simulink model "simplified_sim_for_linearize"  (R2024b)
settings: Solver=VariableStepAuto  StartTime=0.0  StopTime=15  FixedStep=0.05  MaxStep=0.2  RelTol=1e-3
values from neighbouring files (symbols this model uses):
  AfoilA = 0.046    [model_parameters.m]
  AfoilFP = 0.048    [model_parameters.m]
  AfoilFS = 0.048    [model_parameters.m]
  alpha0012 = data0012(:,1)    [model_parameters.m]
  alpha63412wing = data63412wing(:,1)    [model_parameters.m]
  cd0012 = data0012(:,3)    [model_parameters.m]
  cdi63412wing = data63412wing(:,4)    [model_parameters.m]
  cdv63412wing = data63412wing(:,5)    [model_parameters.m]
  cl63412wing = data63412wing(:,3)    [model_parameters.m]
  cm63412wing = data63412wing(:,9)    [model_parameters.m]
  csA = 0.1    [model_parameters.m]
  csF = 0.08    [model_parameters.m]
  foilA_ARM = [-dxa, dya, dza]    [model_parameters.m]
  foilFP_ARM = [dxf, -dyf, dzf]    [model_parameters.m]
  foilFS_ARM = [dxf, dyf, dzf]    [model_parameters.m]
  g = 9.81    [model_parameters.m]
  LAd = 0.08*pi*(0.8)^3/64    (= 0.0020106192983)    [model_parameters.m]
  LFPd = integral(fpint, foilFP_ARM(2)-0.4, foilFP_ARM(2)+0.4)    [model_parameters.m]
  LFSd = integral(fsint, foilFS_ARM(2)-0.4, foilFS_ARM(2)+0.4)    [model_parameters.m]
  M_RB_1 = inv(M_RB)    [dimensionalize_model.m]    (also in model_parameters.m = M_RB^(-1))
  MAC_A = 0.08    [model_parameters.m]
  MAC_FP = 0.08    [model_parameters.m]
  MAC_FS = 0.08    [model_parameters.m]
  mass = 215    [dimensionalize_model.m]    (also in model_parameters.m)
  propwake = 0.05    [model_parameters.m]
  r_g = [0; 0; 0]    [dimensionalize_model.m]    (also in model_parameters.m = [xg, yg, zg])
  rho = 1024.8    [model_parameters.m]
  spanA = 0.76    [model_parameters.m]
  spanFP = 0.76    [model_parameters.m]
  spanFS = 0.76    [model_parameters.m]
  tA = 0.12*0.08    (= 0.0096)    [model_parameters.m]
  tFP = 0.12*0.08    (= 0.0096)    [model_parameters.m]
  tFS = 0.12*0.08    (= 0.0096)    [model_parameters.m]
  usted = 7    [model_parameters.m]
  wagC1 = 0.165    [model_parameters.m]
  wagC2 = 0.335    [model_parameters.m]
  wage1 = 0.0455*(usted/(MAC_FP/2))    (= 7.9625)    [model_parameters.m]
  wage2 = 0.3*(usted/(MAC_FP/2))    (= 52.5)    [model_parameters.m]
  zpr = dza    (= 0.96)    [model_parameters.m]
undefined symbols (not defined in the file or in its folder): magnitude
libraries: mssSimulink x11, matrix_library x3, simulink_extras x3
(part 1 of 2)
settings Model: PauseTimes=3  SnapshotInterval=1  Creator=jskounakis  LastModifiedBy=jskounakis
settings DataIOCC: ExternalInput=getinputstruct(spec1)  InitialState=getstatestruct(spec1)
settings OptimizationCC: ReuseModelBlockBuffer=off
settings RTWCC: GPUComputeCapability=3.5

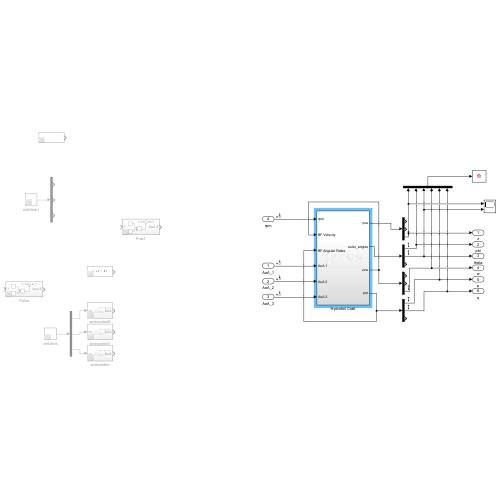
[thumbnail: Simulink's stored preview of the top-level diagram]
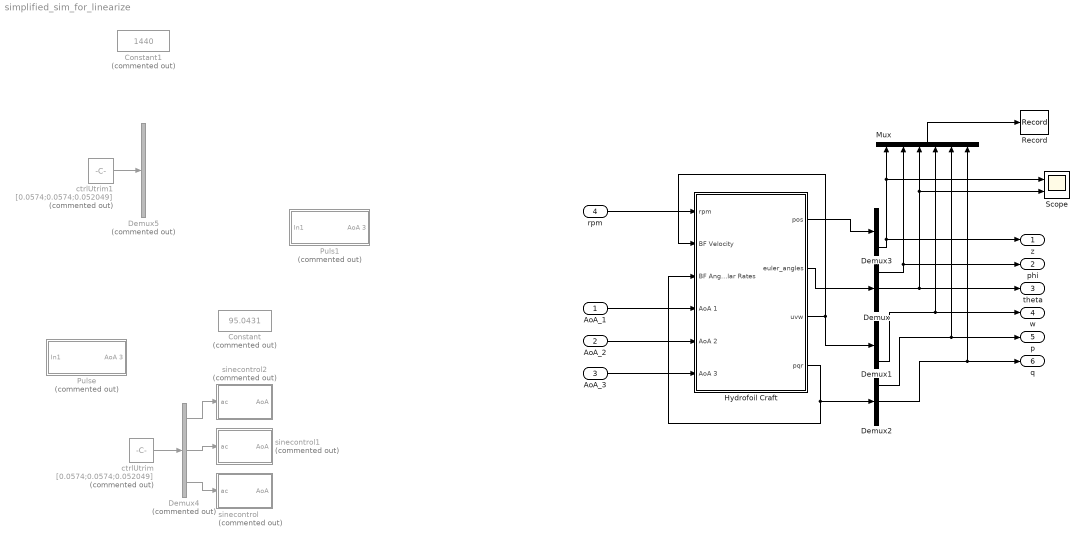
== system simplified_sim_for_linearize ==
  AoA_1 : Inport
  AoA_2 : Inport  Port=2
  AoA_3 : Inport  Port=3
  rpm : Inport  Port=4
  Constant : Constant  Commented=on  Value=95.0431
  Constant1 : Constant  Commented=on  Value=1440
  Demux{,1..3} (4 alike) : Demux  Outputs=3
  Demux4 : Demux  Commented=on  Outputs=3
  Demux5 : Demux  Commented=on  Outputs=3
  Hydrofoil Craft : Subsystem
  Mux : Mux  Inputs=6
  Puls1 : Subsystem  Commented=on
  Pulse : Subsystem  Commented=on
  Record : Record  FileSettingsInternal="{\"entries\":[{\"content\":{\"excelSettings\":{\"content\":{},\"type\":\"Streamout.ExcelSettings\"}},\"type\":\"Streamout.FileSettingStorage\",\"uuid\":\"\"}],\"packageUris\":[\"http:\\/\\/schema.mathworks.com\\/mf0\\/streamout_blocks\\/R2020a\"],\"version\":\"1.0\"}"  Layout=[1 1]  SignalsInternal="{\"entries\":[{\"content\":{\"signals\":[{\"content\":{\"blockPath\":[],\"dimensions\":[6],\"domain\":\"\",\"hasChildren\":true,\"lineColor\":\"#fe330a\",\"lineWidth\":2,\"port\":1,\"signalID\":1,\"signalName\":\"Mux\"},\"type\":\"RecordBlkView.Signal\",\"uuid\":\"\"},{\"content\":{\"blockPath\":[],\"channel\":[1],\"dimensions\":[6],\"domain\":\"\",\"lineColor\":\"#ff6929\",\"lineWidth\":2,\"parentID\":1,\"plots\":[ 1, 27 ],\"port\":1,\"signalID\":2,\"signalName\":\"Mux\"},\"type\":\"RecordBlkView.Signal\",\"uuid\":\"\"},{\"content\":{\"blockPath\":[],\"channel\":[2],\"dimensions\":[6],\"domain\":\"\",\"lineColor\":\"#b746ff\",\"lineWidth\":2,\"parentID\":1,\"plots\":[ 1 ],\"port\":1,\"signalID\":3,\"signalName\":\"Mux\"},\"type\":\"RecordBlkView.Signal\",\"uuid\":\"\"},{\"content\":{\"blockPath\":[],\"channel\":[3],\"dimensions\":[6],\"domain\":\"\",\"lineColor\":\"#64d413\",\"lineWidth\":2,\"parentID\":1,\"plots\":[ 1, 27 ],\"port\":1,\"signalID\":4,\"signalName\":\"Mux\"},\"type\":\"RecordBlkView.Signal\",\"uuid\":\"\"},{\"content\":{\"blockPath\":[],\"channel\":[4],\"dimensions\":[6],\"domain\":\"\",\"lineColor\":\"#ff13a6\",\"lineWidth\":2,\"parentID\":1,\"plots\":[ 1 ],\"port\":1,\"signalID\":5,\"signalName\":\"Mux\"},\"type\":\"RecordBlkView.Signal\",\"uuid\":\"\"},{\"content\":{\"blockPath\":[],\"channel\":[5],\"dimensions\":[6],\"domain\":\"\",\"lineColor\":\"#ff6929\",\"lineWidth\":2,\"parentID\":1,\"plots\":[ 1 ],\"port\":1,\"signalID\":6,\"signalName\":\"Mux\"},\"type\":\"RecordBlkView.Signal\",\"uuid\":\"\"},{\"content\":{\"blockPath\":[],\"channel\":[6],\"dimensions\":[6],\"domain\":\"\",\"lineColor\":\"#ff6929\",\"lineWidth\":2,\"parentID\":1,\"port\":1,\"signalID\":7,\"signalName\":\"Mux\"},\"type\":\"RecordBlkView.Signal\",\"uuid\":\"\"}]},\"type\":\"RecordBlkView.InputSignals\",\"uuid\":\"\"}],\"packageUris\":[\"http:\\/\\/schema.mathworks.com\\/mf0\\/streamout_blocks\\/R2020a\"],\"version\":\"1.0\"}"  VisualizationBindings="{\"sparklinesplugin\":{\"info\":[{\"bindingParametersList\":[],\"subplotID\":1}]}}"
  Scope : Scope  NumInputPorts=2
  ctrlUtrim : Constant  Commented=on  Value=[0.0574;0.0574;0.052049]
  ctrlUtrim1 : Constant  Commented=on  Value=[0.0574;0.0574;0.052049]
  sinecontrol : Subsystem  Commented=on
  sinecontrol1 : Subsystem  Commented=on
  sinecontrol2 : Subsystem  Commented=on
  z : Outport
  phi : Outport  Port=2
  theta : Outport  Port=3
  w : Outport  Port=4
  p : Outport  Port=5
  q : Outport  Port=6
  wires:
  Hydrofoil Craft/3(uvw) -> Demux1/1, Hydrofoil Craft/2(BF Velocity)
  Hydrofoil Craft/2(euler_angles) -> Demux/1
  Hydrofoil Craft/4(pqr) -> Hydrofoil Craft/3(BF Angular Rates), Demux2/1
  Hydrofoil Craft/1(pos) -> Demux3/1
  Demux3/3 -> Mux/1, Scope/1, z/1
  Demux/1 -> Mux/2, phi/1
  Demux/2 -> theta/1, Scope/2, Mux/3
  Demux1/3 -> Mux/4, w/1
  Demux2/2 -> Mux/6, q/1
  Demux2/1 -> Mux/5, p/1
  ctrlUtrim/1 -> Demux4/1
  ctrlUtrim1/1 -> Demux5/1
  Demux4/2 -> sinecontrol1/1(ac)
  Demux4/1 -> sinecontrol2/1(ac)
  Demux4/3 -> sinecontrol/1(ac)
  Mux/1 -> Record/1
  rpm/1 -> Hydrofoil Craft/1(rpm)
  AoA_1/1 -> Hydrofoil Craft/4(AoA 1)
  AoA_2/1 -> Hydrofoil Craft/5(AoA 2)
  AoA_3/1 -> Hydrofoil Craft/6(AoA 3)

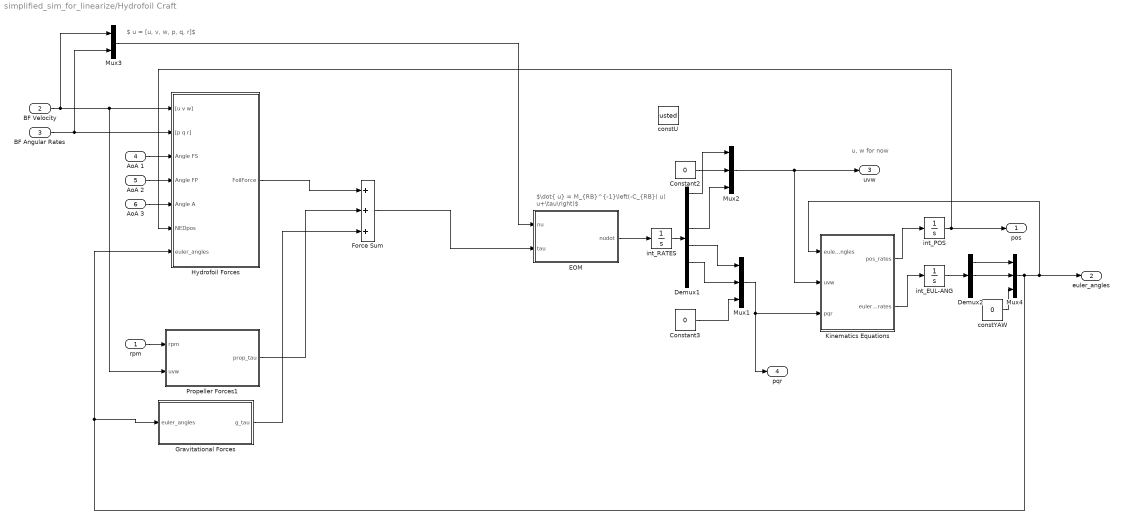
== system simplified_sim_for_linearize/Hydrofoil Craft ==
  note: $\nu = [u, v, w, p, q, r]$
  note: $\dot{\nu} = M_{RB}^{-1}\left(-C_{RB}(\nu)\nu+\tau\right)$
  note: u, w for now
  rpm : Inport
  BF Velocity : Inport  Port=2
  BF Angular Rates : Inport  Port=3
  AoA 1 : Inport  Port=4
  AoA 2 : Inport  Port=5
  AoA 3 : Inport  Port=6
  Constant2 : Constant  Value=0
  Constant3 : Constant  Value=0
  Demux1 : Demux  Outputs=6
  Demux2 : Demux  Outputs=3
  EOM : Subsystem
  Force Sum : Sum  Inputs=+++
  Gravitational Forces : MATLAB Function  TreatAsAtomicUnit=on
  Hydrofoil Forces : Subsystem
  Kinematics Equations : MATLAB Function  TreatAsAtomicUnit=on
  Mux1 : Mux  Inputs=3
  Mux2 : Mux  Inputs=3
  Mux3 : Mux  Inputs=2
  Mux4 : Mux  Inputs=3
  Propeller Forces1 : Subsystem
  constU : Constant  Value=usted
  constYAW : Constant  Value=0
  int_EUL-ANG : Integrator  InitialCondition=[0;0;0]
  int_POS : Integrator  InitialCondition=[0;0;-0.3]
  int_RATES : Integrator  InitialCondition=[usted;0;0;0;0;0]
  pos : Outport
  euler_angles : Outport  Port=2
  uvw : Outport  Port=3
  pqr : Outport  Port=4
  wires:
  BF Angular Rates/1 -> Mux3/2, Hydrofoil Forces/2("[p q r]")
  BF Velocity/1 -> Mux3/1, Propeller Forces1/2(uvw), Hydrofoil Forces/1("[u v w]")
  int_RATES/1 -> Demux1/1
  Mux1/1 -> Kinematics Equations/3(pqr), pqr/1
  Demux1/3 -> Mux2/3
  Demux1/5 -> Mux1/2
  Mux2/1 -> Kinematics Equations/2(uvw), uvw/1
  Kinematics Equations/1(pos_rates) -> int_POS/1
  AoA 2/1 -> Hydrofoil Forces/4(Angle FP)
  AoA 3/1 -> Hydrofoil Forces/5(Angle A)
  AoA 1/1 -> Hydrofoil Forces/3(Angle FS)
  Demux2/1 -> Mux4/1
  Demux2/2 -> Mux4/2
  Mux4/1 -> Gravitational Forces/1(euler_angles), Hydrofoil Forces/7(euler_angles), Kinematics Equations/1(euler_angles), euler_angles/1
  constYAW/1 -> Mux4/3
  int_EUL-ANG/1 -> Demux2/1
  Constant2/1 -> Mux2/2
  rpm/1 -> Propeller Forces1/1(rpm)
  Mux3/1 -> EOM/1(nu)
  EOM/1(nudot) -> int_RATES/1
  Kinematics Equations/2(euler_ang_rates) -> int_EUL-ANG/1
  Demux1/4 -> Mux1/1
  Constant3/1 -> Mux1/3
  int_POS/1 -> pos/1, Hydrofoil Forces/6(NEDpos)
  Demux1/1 -> Mux2/1
  Hydrofoil Forces/1(FoilForce) -> Force Sum/1
  Propeller Forces1/1(prop_tau) -> Force Sum/2
  Gravitational Forces/1(g_tau) -> Force Sum/3
  Force Sum/1 -> EOM/2(tau)

== system simplified_sim_for_linearize/Puls1 ==
  In1 : Inport
  Add1 : Sum
  Step1 : Step  After=0.05  SampleTime=0
  Step2 : Step  Time=1.1  After=-0.05  SampleTime=0
  Sum1 : Sum  Inputs=|++
  AoA 3 : Outport
  wires:
  Step1/1 -> Add1/1
  Add1/1 -> Sum1/2
  In1/1 -> Sum1/1
  Step2/1 -> Add1/2
  Sum1/1 -> AoA 3/1

== system simplified_sim_for_linearize/Pulse ==
  In1 : Inport
  Add1 : Sum
  Step1 : Step  Time=0  SampleTime=0
  Step2 : Step  Time=0.1  After=-1  SampleTime=0
  Sum1 : Sum  Inputs=|++
  AoA 3 : Outport
  wires:
  Step1/1 -> Add1/1
  Add1/1 -> Sum1/2
  In1/1 -> Sum1/1
  Step2/1 -> Add1/2
  Sum1/1 -> AoA 3/1

== system simplified_sim_for_linearize/sinecontrol ==
  ac : Inport
  Clock : Clock
  Product : Product
  Sine Wave Function : Sin  TimeSource=Use external signal  Amplitude=0.0523599*1.5  Frequency=4*pi  SampleTime=0
  Sum : Sum  Inputs=|++
  on : Step  Time=0  SampleTime=0
  AoA : Outport
  wires:
  Clock/1 -> Sine Wave Function/1
  on/1 -> Product/1
  Sine Wave Function/1 -> Product/2
  Product/1 -> Sum/2
  ac/1 -> Sum/1
  Sum/1 -> AoA/1

== system simplified_sim_for_linearize/sinecontrol1 ==
  ac : Inport
  Clock : Clock
  Product : Product
  Sine Wave Function : Sin  TimeSource=Use external signal  Amplitude=0.0523599  Frequency=4*pi()  SampleTime=0
  Sum : Sum  Inputs=|++
  on : Step  Time=0  SampleTime=0
  AoA : Outport
  wires:
  Clock/1 -> Sine Wave Function/1
  on/1 -> Product/1
  Sine Wave Function/1 -> Product/2
  Product/1 -> Sum/2
  ac/1 -> Sum/1
  Sum/1 -> AoA/1

== system simplified_sim_for_linearize/sinecontrol2 ==
  ac : Inport
  Clock : Clock
  Product : Product
  Sine Wave Function : Sin  TimeSource=Use external signal  Amplitude=0.0523599  Frequency=4*pi()  SampleTime=0
  Sum : Sum  Inputs=|++
  on : Step  Time=0  SampleTime=0
  AoA : Outport
  wires:
  Clock/1 -> Sine Wave Function/1
  on/1 -> Product/1
  Sine Wave Function/1 -> Product/2
  Product/1 -> Sum/2
  ac/1 -> Sum/1
  Sum/1 -> AoA/1

== system simplified_sim_for_linearize/Hydrofoil Craft/EOM ==
  note: $-C_{RB}(\nu)\nu+\tau$
  note: $M_{RB}^{-1}$
  note: Rigid Body Coriolis - Centripetal Matrix
  note: $M_{RB}^{-1}\left(-C_{RB}(\nu)\nu+\tau\right)$
  nu : Inport
  tau : Inport  Port=2
  Add3 : Sum  Inputs=-+
  CRB MATRIX : MATLAB Function  TreatAsAtomicUnit=on
  MRB INVERSE : Constant  Value=M_RB_1
  Product1 : Product  Multiplication=Matrix(*)
  Product2 : Product  Multiplication=Matrix(*)
  nudot : Outport
  wires:
  CRB MATRIX/1(C) -> Product2/1
  nu/1 -> Product2/2, CRB MATRIX/1(nu)
  Add3/1 -> Product1/2
  Product2/1 -> Add3/1
  tau/1 -> Add3/2
  Product1/1 -> nudot/1
  MRB INVERSE/1 -> Product1/1

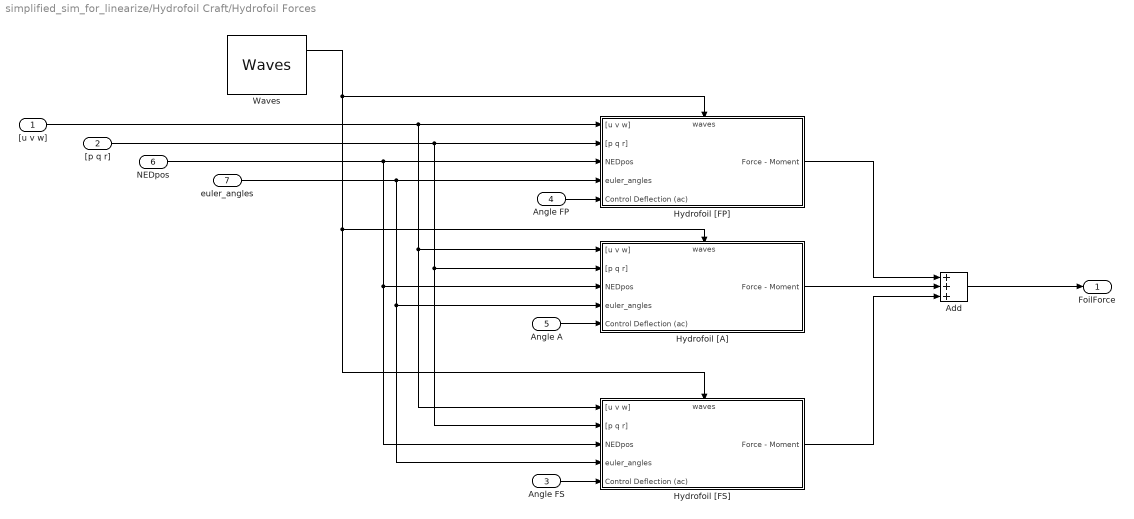
== system simplified_sim_for_linearize/Hydrofoil Craft/Hydrofoil Forces ==
  "[u v w]" : Inport
  "[p q r]" : Inport  Port=2
  Angle FS : Inport  Port=3
  Angle FP : Inport  Port=4
  Angle A : Inport  Port=5
  NEDpos : Inport  Port=6
  euler_angles : Inport  Port=7
  Add : Sum  Inputs=+++
  Hydrofoil [A] : Subsystem
      settings: PortSchema="{\"entries\":[{\"content\":{\"sides\":[{\"content\":{\"connectorIds\":[\"In1\",\"In2\",\"In3\",\"In4\",\"In5\"]},\"type\":\"ConnectorPlacement.EquallySpacedRectSide\",\"uuid\":\"677cb1e4-b507-48e0-bf9b-1d4b68d11740\"},{\"content\":{\"connectorIds\":[\"Out1\"],\"side\":\"RIGHT\"},\"type\":\"ConnectorPlacement.EquallySpacedRectSide\",\"uuid\":\"aaee0231-58d5-427f-802b-fd317cb8babc\"},{\"content\":{\"connectorIds\":[\"In6\"],\"side\":\"TOP\"},\"type\":\"ConnectorPlacement.EquallySpacedRectSide\",\"uuid\":\"1e7dce63-7570-4618-9859-1c6c6aa2cc5b\"}]},\"type\":\"ConnectorPlacement.EquallySpacedConnector\",\"uuid\":\"334cd270-f68d-4b91-93d0-e05f7617c880\"}],\"packageUris\":[\"http://schema.mathworks.com/mf0/Connector/R2020b\"],\"version\":\"1.0\"}"
  Hydrofoil [FP] : Subsystem
      settings: PortSchema="{\"entries\":[{\"content\":{\"sides\":[{\"content\":{\"connectorIds\":[\"In1\",\"In2\",\"In3\",\"In4\",\"In5\"]},\"type\":\"ConnectorPlacement.EquallySpacedRectSide\",\"uuid\":\"677cb1e4-b507-48e0-bf9b-1d4b68d11740\"},{\"content\":{\"connectorIds\":[\"Out1\"],\"side\":\"RIGHT\"},\"type\":\"ConnectorPlacement.EquallySpacedRectSide\",\"uuid\":\"aaee0231-58d5-427f-802b-fd317cb8babc\"},{\"content\":{\"connectorIds\":[\"In6\"],\"side\":\"TOP\"},\"type\":\"ConnectorPlacement.EquallySpacedRectSide\",\"uuid\":\"1e7dce63-7570-4618-9859-1c6c6aa2cc5b\"}]},\"type\":\"ConnectorPlacement.EquallySpacedConnector\",\"uuid\":\"334cd270-f68d-4b91-93d0-e05f7617c880\"}],\"packageUris\":[\"http://schema.mathworks.com/mf0/Connector/R2020b\"],\"version\":\"1.0\"}"
  Hydrofoil [FS] : Subsystem
      settings: PortSchema="{\"entries\":[{\"content\":{\"sides\":[{\"content\":{\"connectorIds\":[\"In1\",\"In2\",\"In3\",\"In4\",\"In5\"]},\"type\":\"ConnectorPlacement.EquallySpacedRectSide\",\"uuid\":\"677cb1e4-b507-48e0-bf9b-1d4b68d11740\"},{\"content\":{\"connectorIds\":[\"Out1\"],\"side\":\"RIGHT\"},\"type\":\"ConnectorPlacement.EquallySpacedRectSide\",\"uuid\":\"aaee0231-58d5-427f-802b-fd317cb8babc\"},{\"content\":{\"connectorIds\":[\"In6\"],\"side\":\"TOP\"},\"type\":\"ConnectorPlacement.EquallySpacedRectSide\",\"uuid\":\"1e7dce63-7570-4618-9859-1c6c6aa2cc5b\"}]},\"type\":\"ConnectorPlacement.EquallySpacedConnector\",\"uuid\":\"334cd270-f68d-4b91-93d0-e05f7617c880\"}],\"packageUris\":[\"http://schema.mathworks.com/mf0/Connector/R2020b\"],\"version\":\"1.0\"}"
  Waves : mssSimulink/Environment/Waves/Waves  spectrum_type=Predefined waves  disp_flag=on  plot_spectrum=off  plot_realization=off  hs=0.5  omega_peak=1  psi_mean=0  gamma=-1  spread=2  depth=inf  nfreq=20  ndir=10  energylim=0.005  freq_cutoff=3  dir_cutoff=0  rand_seed=321  rand_freq=on  rand_dir=on  Zeta_a=0  Omega=0  Phase=0  Wavenum=0  Psi=pi()
  FoilForce : Outport
  wires:
  Angle A/1 -> Hydrofoil [A]/5(Control Deflection (ac))
  Angle FP/1 -> Hydrofoil [FP]/5(Control Deflection (ac))
  "[u v w]"/1 -> Hydrofoil [FS]/1("[u v w]"), Hydrofoil [A]/1("[u v w]"), Hydrofoil [FP]/1("[u v w]")
  "[p q r]"/1 -> Hydrofoil [FP]/2("[p q r]"), Hydrofoil [FS]/2("[p q r]"), Hydrofoil [A]/2("[p q r]")
  Hydrofoil [FP]/1(Force - Moment) -> Add/1
  Add/1 -> FoilForce/1
  euler_angles/1 -> Hydrofoil [FP]/4(euler_angles), Hydrofoil [FS]/4(euler_angles), Hydrofoil [A]/4(euler_angles)
  NEDpos/1 -> Hydrofoil [FP]/3(NEDpos), Hydrofoil [FS]/3(NEDpos), Hydrofoil [A]/3(NEDpos)
  Hydrofoil [A]/1(Force - Moment) -> Add/2
  Angle FS/1 -> Hydrofoil [FS]/5(Control Deflection (ac))
  Hydrofoil [FS]/1(Force - Moment) -> Add/3
  Waves/1 -> Hydrofoil [FS]/6(waves), Hydrofoil [A]/6(waves), Hydrofoil [FP]/6(waves)

== system simplified_sim_for_linearize/Hydrofoil Craft/Propeller Forces1 ==
  rpm : Inport
  uvw : Inport  Port=2
  Gain : Gain  Gain=1/60
  Mux : Mux  Inputs=6
  Open-water propeller characteristics : mssSimulink/Modelling/Propulsion/Open-water propeller characteristics  Par_Thruster_D=propD  Par_Thruster_Ktp=propKtp  Par_Thruster_Kqp=propKqp  Par_Thruster_reverse_reduction=0.8  Glob_rhow=rho
  Product : Product
  Product1 : Product
  Propeller Arm : Constant  Value=zpr
  Selector : Selector  InputPortWidth=3  IndexOptions=Index vector (dialog)  Indices=[1]  OutputSizes=1
  wake : Constant  Value=1-propwake
  prop_tau : Outport
  wires:
  Propeller Arm/1 -> Product/1
  Product/1 -> Mux/5
  wake/1 -> Product1/1
  Product1/1 -> Open-water propeller characteristics/2
  rpm/1 -> Gain/1
  Gain/1 -> Open-water propeller characteristics/1
  Open-water propeller characteristics/1 -> Mux/1, Product/2
  uvw/1 -> Selector/1
  Selector/1 -> Product1/2
  Mux/1 -> prop_tau/1

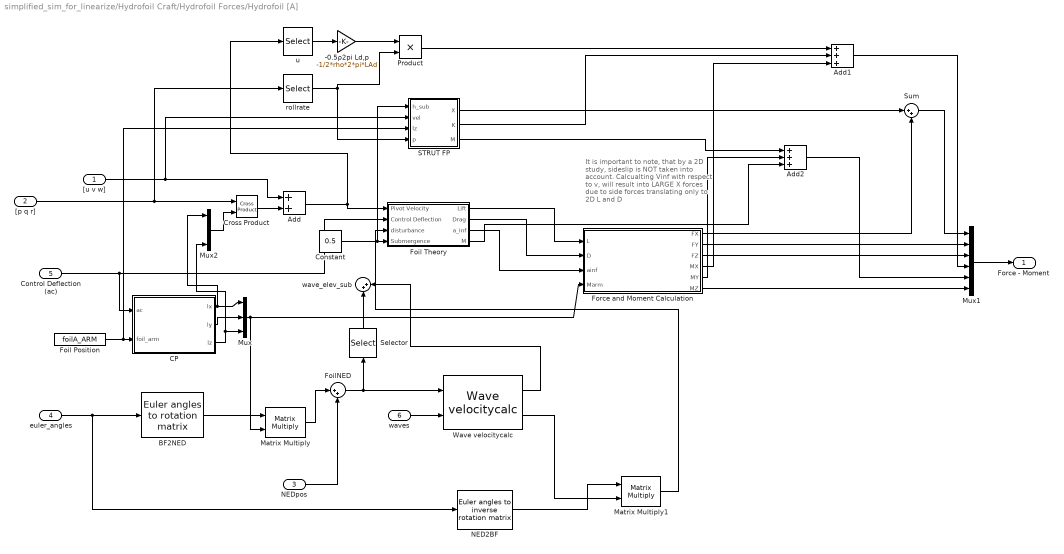
== system simplified_sim_for_linearize/Hydrofoil Craft/Hydrofoil Forces/Hydrofoil [A] ==
  note: It is important to note,
      | that by a 2D study, sideslip
      | is NOT taken into account.
      | Calcualting Vinf with respect
      | to v, will result into LARGE X
      | forces due to side forces translating
      | only to 2D L and D
  "[u v w]" : Inport
  "[p q r]" : Inport  Port=2
  NEDpos : Inport  Port=3
  euler_angles : Inport  Port=4
  Control Deflection (ac) : Inport  Port=5
  waves : Inport  Port=6
  -0.5ρ2pi Ld,p : Gain  Gain=-1/2*rho*2*pi*LAd
  Add : Sum
  Add1 : Sum  Inputs=+++
  Add2 : Sum  Inputs=+++
  BF2NED : mssSimulink/Modelling/Kinematics/Euler angles to rotation matrix
  CP : MATLAB Function  TreatAsAtomicUnit=on
  Constant : Constant  Value=0.5
  Cross Product : matrix_library/Cross Product
  Foil Position : Constant  Value=foilA_ARM
  Foil Theory : Subsystem
  FoilNED : Sum  Inputs=|++
  Force and Moment Calculation : MATLAB Function  TreatAsAtomicUnit=on
  Matrix Multiply : Product  Multiplication=Matrix(*)
  Matrix Multiply1 : Product  Multiplication=Matrix(*)
  Mux : Mux  Inputs=3
  Mux1 : Mux  Inputs=6
  Mux2 : Mux  Inputs=3
  NED2BF : mssSimulink/Modelling/Kinematics/Euler angles to inverse rotation matrix
  Product : Product
  STRUT FP : Subsystem
  Selector : Selector  InputPortWidth=3  IndexOptions=Index vector (dialog)  Indices=[3]  OutputSizes=1
  Sum : Sum  Inputs=|++
  Wave velocitycalc : mssSimulink/Environment/Waves/Wave velocitycalc
  rollrate : Selector  InputPortWidth=3  IndexOptions=Index vector (dialog)  Indices=[1]  OutputSizes=1
  u : Selector  InputPortWidth=3  IndexOptions=Index vector (dialog)  Indices=[1]  OutputSizes=1
  wave_elev_sub : Sum  Inputs=|++
  Force - Moment : Outport
  wires:
  "[u v w]"/1 -> STRUT FP/2(vel), Add/1
  Cross Product/1 -> Add/2
  "[p q r]"/1 -> rollrate/1, Cross Product/1
  Control Deflection (ac)/1 -> Foil Theory/2(Control Deflection), CP/1(ac)
  CP/1(lx) -> Mux2/1, Mux/1
  CP/2(ly) -> Mux/2
  CP/3(lz) -> Mux2/3, Mux/3
  Mux/1 -> Matrix Multiply/2, Force and Moment Calculation/4(Marm)
  Force and Moment Calculation/2(FY) -> Mux1/2
  Force and Moment Calculation/3(FZ) -> Mux1/3
  Force and Moment Calculation/6(MZ) -> Mux1/6
  Mux1/1 -> Force - Moment/1
  Foil Position/1 -> STRUT FP/3(lz), CP/2(foil_arm)
  euler_angles/1 -> NED2BF/1, BF2NED/1
  Add/1 -> u/1, Foil Theory/1(Pivot Velocity)
  Foil Theory/1(Lift) -> Force and Moment Calculation/1(L)
  Foil Theory/2(Drag) -> Force and Moment Calculation/2(D)
  Foil Theory/3(a_inf) -> Force and Moment Calculation/3(ainf)
  BF2NED/1 -> Matrix Multiply/1
  Matrix Multiply/1 -> FoilNED/1
  NEDpos/1 -> FoilNED/2
  FoilNED/1 -> Wave velocitycalc/1, Selector/1
  Sum/1 -> Mux1/1
  Force and Moment Calculation/1(FX) -> Sum/2
  STRUT FP/1(X) -> Sum/1
  STRUT FP/3(M) -> Add2/1
  Force and Moment Calculation/5(MY) -> Add2/2
  Add2/1 -> Mux1/5
  STRUT FP/2(K) -> Add1/2
  Force and Moment Calculation/4(MX) -> Add1/3
  Add1/1 -> Mux1/4
  Mux2/1 -> Cross Product/2
  rollrate/1 -> Product/2, STRUT FP/4(p)
  -0.5ρ2pi Ld,p/1 -> Product/1
  u/1 -> -0.5ρ2pi Ld,p/1
  Product/1 -> Add1/1
  Wave velocitycalc/1 -> wave_elev_sub/2
  Wave velocitycalc/2 -> Matrix Multiply1/2
  NED2BF/1 -> Matrix Multiply1/1
  Selector/1 -> wave_elev_sub/1
  waves/1 -> Wave velocitycalc/2
  Matrix Multiply1/1 -> Foil Theory/3(disturbance)
  Constant/1 -> STRUT FP/1(h_sub), Foil Theory/4(Submergence)
  Foil Theory/4(M) -> Add2/3

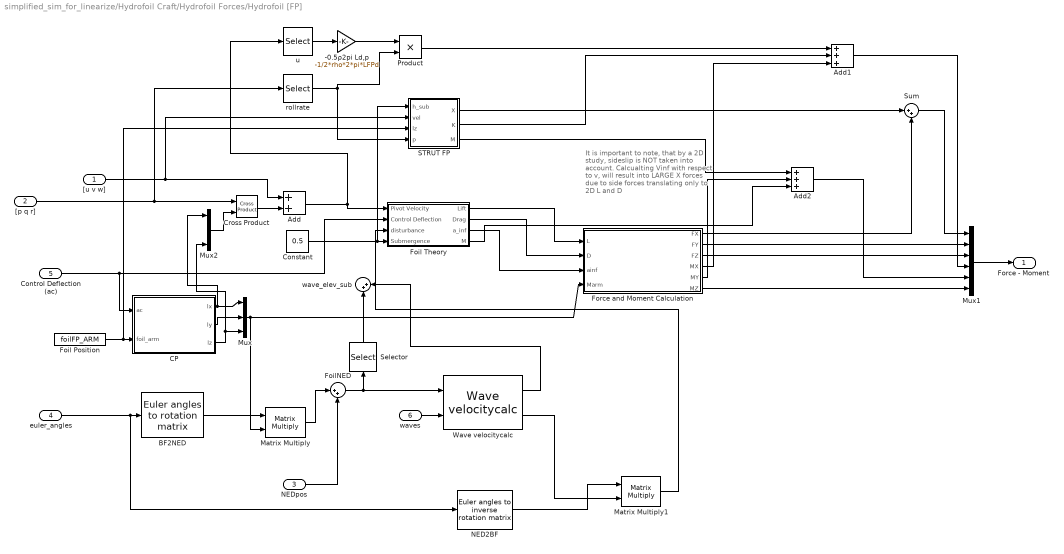
== system simplified_sim_for_linearize/Hydrofoil Craft/Hydrofoil Forces/Hydrofoil [FP] ==
  note: It is important to note,
      | that by a 2D study, sideslip
      | is NOT taken into account.
      | Calcualting Vinf with respect
      | to v, will result into LARGE X
      | forces due to side forces translating
      | only to 2D L and D
  "[u v w]" : Inport
  "[p q r]" : Inport  Port=2
  NEDpos : Inport  Port=3
  euler_angles : Inport  Port=4
  Control Deflection (ac) : Inport  Port=5
  waves : Inport  Port=6
  -0.5ρ2pi Ld,p : Gain  Gain=-1/2*rho*2*pi*LFPd
  Add : Sum
  Add1 : Sum  Inputs=+++
  Add2 : Sum  Inputs=+++
  BF2NED : mssSimulink/Modelling/Kinematics/Euler angles to rotation matrix
  CP : MATLAB Function  TreatAsAtomicUnit=on
  Constant : Constant  Value=0.5
  Cross Product : matrix_library/Cross Product
  Foil Position : Constant  Value=foilFP_ARM
  Foil Theory : Subsystem
  FoilNED : Sum  Inputs=|++
  Force and Moment Calculation : MATLAB Function  TreatAsAtomicUnit=on
  Matrix Multiply : Product  Multiplication=Matrix(*)
  Matrix Multiply1 : Product  Multiplication=Matrix(*)
  Mux : Mux  Inputs=3
  Mux1 : Mux  Inputs=6
  Mux2 : Mux  Inputs=3
  NED2BF : mssSimulink/Modelling/Kinematics/Euler angles to inverse rotation matrix
  Product : Product
  STRUT FP : Subsystem
  Selector : Selector  InputPortWidth=3  IndexOptions=Index vector (dialog)  Indices=[3]  OutputSizes=1
  Sum : Sum  Inputs=|++
  Wave velocitycalc : mssSimulink/Environment/Waves/Wave velocitycalc
  rollrate : Selector  InputPortWidth=3  IndexOptions=Index vector (dialog)  Indices=[1]  OutputSizes=1
  u : Selector  InputPortWidth=3  IndexOptions=Index vector (dialog)  Indices=[1]  OutputSizes=1
  wave_elev_sub : Sum  Inputs=|++
  Force - Moment : Outport
  wires:
  "[u v w]"/1 -> STRUT FP/2(vel), Add/1
  Cross Product/1 -> Add/2
  "[p q r]"/1 -> rollrate/1, Cross Product/1
  Control Deflection (ac)/1 -> Foil Theory/2(Control Deflection), CP/1(ac)
  CP/1(lx) -> Mux2/1, Mux/1
  CP/2(ly) -> Mux/2
  CP/3(lz) -> Mux2/3, Mux/3
  Mux/1 -> Matrix Multiply/2, Force and Moment Calculation/4(Marm)
  Force and Moment Calculation/2(FY) -> Mux1/2
  Force and Moment Calculation/3(FZ) -> Mux1/3
  Force and Moment Calculation/6(MZ) -> Mux1/6
  Mux1/1 -> Force - Moment/1
  Foil Position/1 -> STRUT FP/3(lz), CP/2(foil_arm)
  euler_angles/1 -> NED2BF/1, BF2NED/1
  Add/1 -> u/1, Foil Theory/1(Pivot Velocity)
  Foil Theory/1(Lift) -> Force and Moment Calculation/1(L)
  Foil Theory/2(Drag) -> Force and Moment Calculation/2(D)
  Foil Theory/3(a_inf) -> Force and Moment Calculation/3(ainf)
  BF2NED/1 -> Matrix Multiply/1
  Matrix Multiply/1 -> FoilNED/1
  NEDpos/1 -> FoilNED/2
  FoilNED/1 -> Wave velocitycalc/1, Selector/1
  Sum/1 -> Mux1/1
  Force and Moment Calculation/1(FX) -> Sum/2
  STRUT FP/1(X) -> Sum/1
  STRUT FP/3(M) -> Add2/1
  Force and Moment Calculation/5(MY) -> Add2/2
  Add2/1 -> Mux1/5
  STRUT FP/2(K) -> Add1/2
  Force and Moment Calculation/4(MX) -> Add1/3
  Add1/1 -> Mux1/4
  Mux2/1 -> Cross Product/2
  rollrate/1 -> Product/2, STRUT FP/4(p)
  -0.5ρ2pi Ld,p/1 -> Product/1
  u/1 -> -0.5ρ2pi Ld,p/1
  Product/1 -> Add1/1
  waves/1 -> Wave velocitycalc/2
  Wave velocitycalc/1 -> wave_elev_sub/2
  NED2BF/1 -> Matrix Multiply1/1
  Wave velocitycalc/2 -> Matrix Multiply1/2
  Selector/1 -> wave_elev_sub/1
  Matrix Multiply1/1 -> Foil Theory/3(disturbance)
  Constant/1 -> STRUT FP/1(h_sub), Foil Theory/4(Submergence)
  Foil Theory/4(M) -> Add2/3

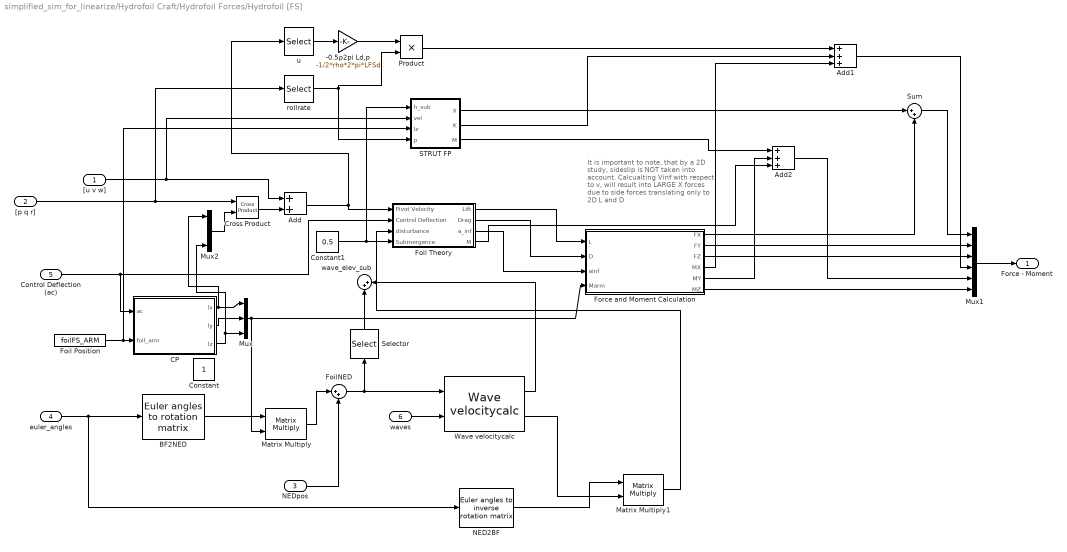
== system simplified_sim_for_linearize/Hydrofoil Craft/Hydrofoil Forces/Hydrofoil [FS] ==
  note: It is important to note,
      | that by a 2D study, sideslip
      | is NOT taken into account.
      | Calcualting Vinf with respect
      | to v, will result into LARGE X
      | forces due to side forces translating
      | only to 2D L and D
  "[u v w]" : Inport
  "[p q r]" : Inport  Port=2
  NEDpos : Inport  Port=3
  euler_angles : Inport  Port=4
  Control Deflection (ac) : Inport  Port=5
  waves : Inport  Port=6
  -0.5ρ2pi Ld,p : Gain  Gain=-1/2*rho*2*pi*LFSd
  Add : Sum
  Add1 : Sum  Inputs=+++
  Add2 : Sum  Inputs=+++
  BF2NED : mssSimulink/Modelling/Kinematics/Euler angles to rotation matrix
  CP : MATLAB Function  TreatAsAtomicUnit=on
  Constant : Constant
  Constant1 : Constant  Value=0.5
  Cross Product : matrix_library/Cross Product
  Foil Position : Constant  Value=foilFS_ARM
  Foil Theory : Subsystem
  FoilNED : Sum  Inputs=|++
  Force and Moment Calculation : MATLAB Function  TreatAsAtomicUnit=on
  Matrix Multiply : Product  Multiplication=Matrix(*)
  Matrix Multiply1 : Product  Multiplication=Matrix(*)
  Mux : Mux  Inputs=3
  Mux1 : Mux  Inputs=6
  Mux2 : Mux  Inputs=3
  NED2BF : mssSimulink/Modelling/Kinematics/Euler angles to inverse rotation matrix
  Product : Product
  STRUT FP : Subsystem
  Selector : Selector  InputPortWidth=3  IndexOptions=Index vector (dialog)  Indices=[3]  OutputSizes=1
  Sum : Sum  Inputs=|++
  Wave velocitycalc : mssSimulink/Environment/Waves/Wave velocitycalc
  rollrate : Selector  InputPortWidth=3  IndexOptions=Index vector (dialog)  Indices=[1]  OutputSizes=1
  u : Selector  InputPortWidth=3  IndexOptions=Index vector (dialog)  Indices=[1]  OutputSizes=1
  wave_elev_sub : Sum  Inputs=|++
  Force - Moment : Outport
  wires:
  "[u v w]"/1 -> STRUT FP/2(vel), Add/1
  Cross Product/1 -> Add/2
  "[p q r]"/1 -> rollrate/1, Cross Product/1
  Control Deflection (ac)/1 -> Foil Theory/2(Control Deflection), CP/1(ac)
  CP/1(lx) -> Mux2/1, Mux/1
  CP/2(ly) -> Mux/2
  CP/3(lz) -> Mux2/3, Mux/3
  Mux/1 -> Matrix Multiply/2, Force and Moment Calculation/4(Marm)
  Force and Moment Calculation/2(FY) -> Mux1/2
  Force and Moment Calculation/3(FZ) -> Mux1/3
  Force and Moment Calculation/6(MZ) -> Mux1/6
  Mux1/1 -> Force - Moment/1
  Foil Position/1 -> STRUT FP/3(lz), CP/2(foil_arm)
  euler_angles/1 -> NED2BF/1, BF2NED/1
  Add/1 -> u/1, Foil Theory/1(Pivot Velocity)
  Foil Theory/1(Lift) -> Force and Moment Calculation/1(L)
  Foil Theory/2(Drag) -> Force and Moment Calculation/2(D)
  Foil Theory/3(a_inf) -> Force and Moment Calculation/3(ainf)
  BF2NED/1 -> Matrix Multiply/1
  Matrix Multiply/1 -> FoilNED/1
  NEDpos/1 -> FoilNED/2
  FoilNED/1 -> Selector/1, Wave velocitycalc/1
  Sum/1 -> Mux1/1
  Force and Moment Calculation/1(FX) -> Sum/2
  STRUT FP/1(X) -> Sum/1
  STRUT FP/3(M) -> Add2/1
  Force and Moment Calculation/5(MY) -> Add2/2
  Add2/1 -> Mux1/5
  STRUT FP/2(K) -> Add1/2
  Force and Moment Calculation/4(MX) -> Add1/3
  Add1/1 -> Mux1/4
  Mux2/1 -> Cross Product/2
  rollrate/1 -> Product/2, STRUT FP/4(p)
  -0.5ρ2pi Ld,p/1 -> Product/1
  u/1 -> -0.5ρ2pi Ld,p/1
  Product/1 -> Add1/1
  Wave velocitycalc/1 -> wave_elev_sub/2
  Wave velocitycalc/2 -> Matrix Multiply1/2
  NED2BF/1 -> Matrix Multiply1/1
  Selector/1 -> wave_elev_sub/1
  waves/1 -> Wave velocitycalc/2
  Matrix Multiply1/1 -> Foil Theory/3(disturbance)
  Constant1/1 -> STRUT FP/1(h_sub), Foil Theory/4(Submergence)
  Foil Theory/4(M) -> Add2/3

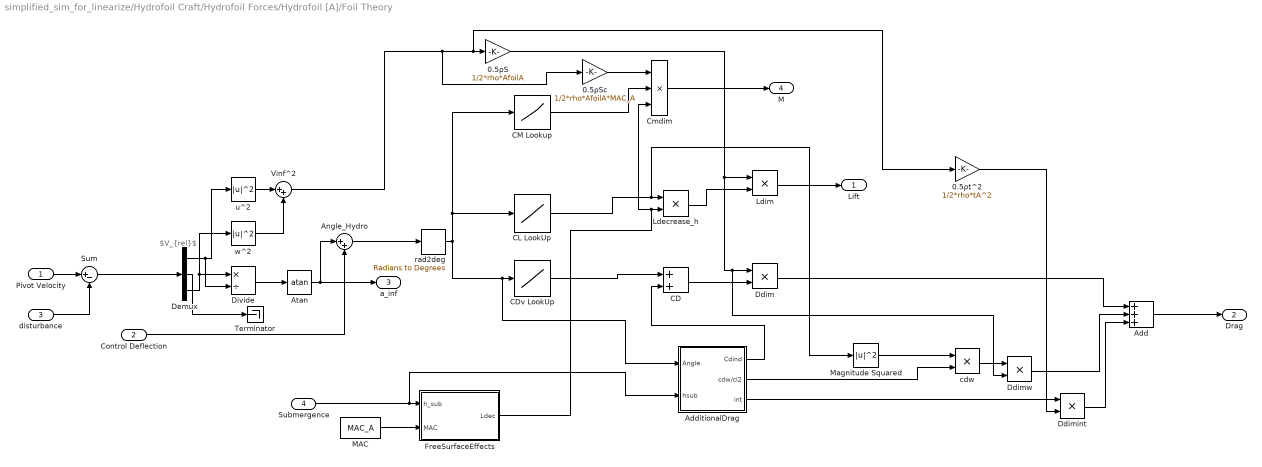
== system simplified_sim_for_linearize/Hydrofoil Craft/Hydrofoil Forces/Hydrofoil [A]/Foil Theory ==
  note: $V_{rel}$
  Pivot Velocity : Inport
  Control Deflection : Inport  Port=2
  disturbance : Inport  Port=3
  Submergence : Inport  Port=4
  0.5ρS : Gain  Gain=1/2*rho*AfoilA
  0.5ρSc : Gain  Gain=1/2*rho*AfoilA*MAC_A
  0.5ρt^2 : Gain  Gain=1/2*rho*tA^2
  Add : Sum  Inputs=+++
  AdditionalDrag : Subsystem
  Angle_Hydro : Sum  Inputs=|++
  Atan : Trigonometry  Operator=atan
  CD : Sum
  CDv LookUp : Lookup_n-D  NumberOfTableDimensions=1  BreakpointsForDimension1=alpha63412wing  Table=cdv63412wing  InternalRulePriority=Speed  RndMeth=Simplest
  CL LookUp : Lookup_n-D  NumberOfTableDimensions=1  BreakpointsForDimension1=alpha63412wing  Table=cl63412wing  InternalRulePriority=Speed  RndMeth=Simplest
  CM Lookup : Lookup_n-D  NumberOfTableDimensions=1  BreakpointsForDimension1=alpha63412wing  Table=cm63412wing  InternalRulePriority=Speed  RndMeth=Simplest
  Cmdim : Product  Inputs=3
  Ddim : Product
  Ddimint : Product
  Ddimw : Product
  Demux : Demux  Outputs=3
  Divide : Product  Inputs=*/
  FreeSurfaceEffects : MATLAB Function  TreatAsAtomicUnit=on
  Ldecrease_h : Product
  Ldim : Product
  MAC : Constant  Value=MAC_A
  Magnitude Squared : Math  Operator=magnitude^2
  Sum : Sum  Inputs=|+-
  Terminator : Terminator
  Vinf^2 : Sum  Inputs=|++
  cdw : Product
  rad2deg : simulink_extras/Transformations/Radians to Degrees
  u^2 : Math  Operator=magnitude^2
  w^2 : Math  Operator=magnitude^2
  Lift : Outport
  Drag : Outport  Port=2
  a_inf : Outport  Port=3
  M : Outport  Port=4
  wires:
  rad2deg/1 -> AdditionalDrag/1(Angle), CDv LookUp/1, CM Lookup/1, CL LookUp/1
  Demux/3 -> w^2/1, Divide/1
  Vinf^2/1 -> 0.5ρSc/1, 0.5ρt^2/1, 0.5ρS/1
  w^2/1 -> Vinf^2/2
  Demux/1 -> u^2/1, Divide/2
  Atan/1 -> a_inf/1, Angle_Hydro/1
  0.5ρS/1 -> Ddimw/2, Ddim/1, Ldim/1
  u^2/1 -> Vinf^2/1
  Divide/1 -> Atan/1
  Control Deflection/1 -> Angle_Hydro/2
  Demux/2 -> Terminator/1
  Ldim/1 -> Lift/1
  Sum/1 -> Demux/1
  disturbance/1 -> Sum/2
  Pivot Velocity/1 -> Sum/1
  Submergence/1 -> AdditionalDrag/2(hsub), FreeSurfaceEffects/1(h_sub)
  MAC/1 -> FreeSurfaceEffects/2(MAC)
  FreeSurfaceEffects/1(Ldec) -> Cmdim/3, Ldecrease_h/2
  CL LookUp/1 -> Magnitude Squared/1, Ldecrease_h/1
  Ldecrease_h/1 -> Ldim/2
  CDv LookUp/1 -> CD/1
  CD/1 -> Ddim/2
  AdditionalDrag/1(Cdind) -> CD/2
  Ddim/1 -> Add/1
  Magnitude Squared/1 -> cdw/1
  AdditionalDrag/2(cdw/cl2) -> cdw/2
  cdw/1 -> Ddimw/1
  Ddimw/1 -> Add/2
  AdditionalDrag/3(int) -> Ddimint/1
  Add/1 -> Drag/1
  0.5ρt^2/1 -> Ddimint/2
  Ddimint/1 -> Add/3
  Angle_Hydro/1 -> rad2deg/1
  0.5ρSc/1 -> Cmdim/1
  CM Lookup/1 -> Cmdim/2
  Cmdim/1 -> M/1

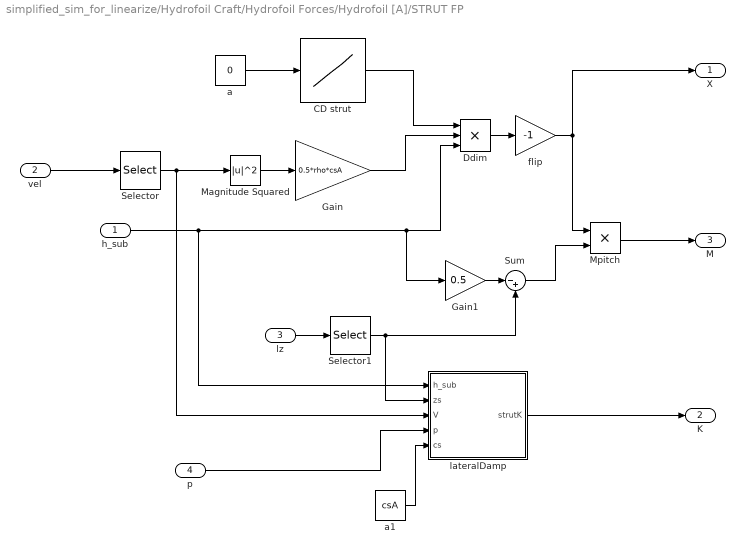
== system simplified_sim_for_linearize/Hydrofoil Craft/Hydrofoil Forces/Hydrofoil [A]/STRUT FP ==
  h_sub : Inport
  vel : Inport  Port=2
  lz : Inport  Port=3
  p : Inport  Port=4
  CD strut : Lookup_n-D  NumberOfTableDimensions=1  BreakpointsForDimension1=alpha0012  Table=cd0012  InternalRulePriority=Speed  RndMeth=Simplest
  Ddim : Product  Inputs=3
  Gain : Gain  Gain=0.5*rho*csA
  Gain1 : Gain  Gain=0.5
  Magnitude Squared : Math  Operator=magnitude^2
  Mpitch : Product
  Selector : Selector  InputPortWidth=3  IndexOptions=Index vector (dialog)  Indices=[1]  OutputSizes=1
  Selector1 : Selector  InputPortWidth=3  IndexOptions=Index vector (dialog)  Indices=[3]  OutputSizes=1
  Sum : Sum  Inputs=|-+
  a : Constant  Value=0
  a1 : Constant  Value=csA
  flip : Gain  Gain=-1
  lateralDamp : MATLAB Function  TreatAsAtomicUnit=on
  X : Outport
  K : Outport  Port=2
  M : Outport  Port=3
  wires:
  vel/1 -> Selector/1
  Selector/1 -> Magnitude Squared/1, lateralDamp/3(V)
  Magnitude Squared/1 -> Gain/1
  a/1 -> CD strut/1
  CD strut/1 -> Ddim/1
  Gain/1 -> Ddim/2
  h_sub/1 -> lateralDamp/1(h_sub), Ddim/3, Gain1/1
  Mpitch/1 -> M/1
  Gain1/1 -> Sum/1
  Sum/1 -> Mpitch/2
  Ddim/1 -> flip/1
  flip/1 -> Mpitch/1, X/1
  lz/1 -> Selector1/1
  Selector1/1 -> lateralDamp/2(zs), Sum/2
  a1/1 -> lateralDamp/5(cs)
  p/1 -> lateralDamp/4(p)
  lateralDamp/1(strutK) -> K/1

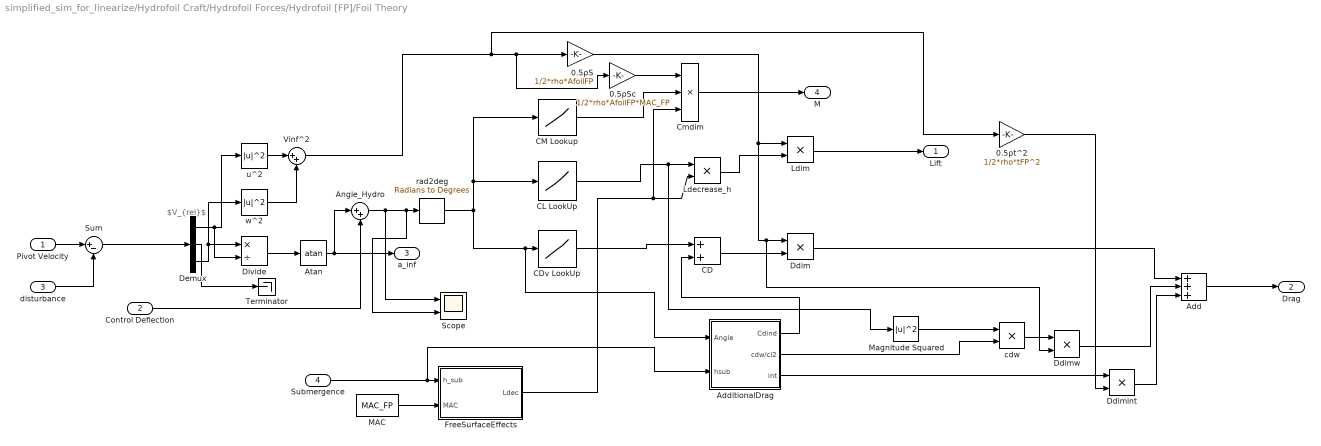
== system simplified_sim_for_linearize/Hydrofoil Craft/Hydrofoil Forces/Hydrofoil [FP]/Foil Theory ==
  note: $V_{rel}$
  Pivot Velocity : Inport
  Control Deflection : Inport  Port=2
  disturbance : Inport  Port=3
  Submergence : Inport  Port=4
  0.5ρS : Gain  Gain=1/2*rho*AfoilFP
  0.5ρSc : Gain  Gain=1/2*rho*AfoilFP*MAC_FP
  0.5ρt^2 : Gain  Gain=1/2*rho*tFP^2
  Add : Sum  Inputs=+++
  AdditionalDrag : Subsystem
  Angle_Hydro : Sum  Inputs=|++
  Atan : Trigonometry  Operator=atan
  CD : Sum
  CDv LookUp : Lookup_n-D  NumberOfTableDimensions=1  BreakpointsForDimension1=alpha63412wing  Table=cdv63412wing  InternalRulePriority=Speed  RndMeth=Simplest
  CL LookUp : Lookup_n-D  NumberOfTableDimensions=1  BreakpointsForDimension1=alpha63412wing  Table=cl63412wing  InternalRulePriority=Speed  RndMeth=Simplest
  CM Lookup : Lookup_n-D  NumberOfTableDimensions=1  BreakpointsForDimension1=alpha63412wing  Table=cm63412wing  InternalRulePriority=Speed  RndMeth=Simplest
  Cmdim : Product  Inputs=3
  Ddim : Product
  Ddimint : Product
  Ddimw : Product
  Demux : Demux  Outputs=3
  Divide : Product  Inputs=*/
  FreeSurfaceEffects : MATLAB Function  TreatAsAtomicUnit=on
  Ldecrease_h : Product
  Ldim : Product
  MAC : Constant  Value=MAC_FP
  Magnitude Squared : Math  Operator=magnitude^2
  Scope : Scope  NumInputPorts=2
  Sum : Sum  Inputs=|+-
  Terminator : Terminator
  Vinf^2 : Sum  Inputs=|++
  cdw : Product
  rad2deg : simulink_extras/Transformations/Radians to Degrees
  u^2 : Math  Operator=magnitude^2
  w^2 : Math  Operator=magnitude^2
  Lift : Outport
  Drag : Outport  Port=2
  a_inf : Outport  Port=3
  M : Outport  Port=4
  wires:
  rad2deg/1 -> AdditionalDrag/1(Angle), CDv LookUp/1, CM Lookup/1, CL LookUp/1
  Demux/3 -> w^2/1, Divide/1
  Vinf^2/1 -> 0.5ρt^2/1, 0.5ρSc/1, 0.5ρS/1
  w^2/1 -> Vinf^2/2
  Demux/1 -> u^2/1, Divide/2
  Atan/1 -> a_inf/1, Angle_Hydro/1
  0.5ρS/1 -> Ddimw/2, Ddim/1, Ldim/1
  u^2/1 -> Vinf^2/1
  Divide/1 -> Atan/1
  Control Deflection/1 -> Angle_Hydro/2
  Demux/2 -> Terminator/1
  Sum/1 -> Demux/1
  disturbance/1 -> Sum/2
  Pivot Velocity/1 -> Sum/1
  Submergence/1 -> AdditionalDrag/2(hsub), FreeSurfaceEffects/1(h_sub)
  MAC/1 -> FreeSurfaceEffects/2(MAC)
  FreeSurfaceEffects/1(Ldec) -> Cmdim/3, Ldecrease_h/2
  CL LookUp/1 -> Ldecrease_h/1, Magnitude Squared/1
  Ldecrease_h/1 -> Ldim/2
  CDv LookUp/1 -> CD/1
  CD/1 -> Ddim/2
  AdditionalDrag/1(Cdind) -> CD/2
  Ddim/1 -> Add/1
  Magnitude Squared/1 -> cdw/1
  AdditionalDrag/2(cdw/cl2) -> cdw/2
  cdw/1 -> Ddimw/1
  Ddimw/1 -> Add/2
  AdditionalDrag/3(int) -> Ddimint/1
  Add/1 -> Drag/1
  0.5ρt^2/1 -> Ddimint/2
  Ddimint/1 -> Add/3
  Ldim/1 -> Lift/1
  Angle_Hydro/1 -> Scope/2, rad2deg/1, Scope/1
  0.5ρSc/1 -> Cmdim/1
  CM Lookup/1 -> Cmdim/2
  Cmdim/1 -> M/1

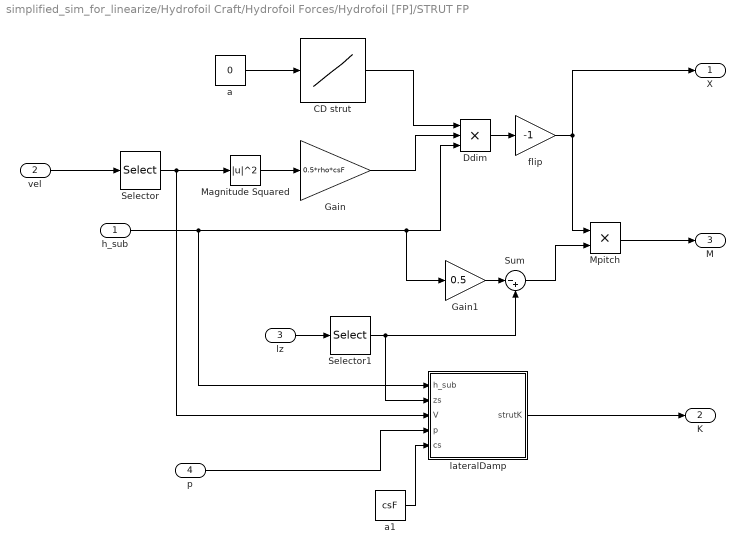
== system simplified_sim_for_linearize/Hydrofoil Craft/Hydrofoil Forces/Hydrofoil [FP]/STRUT FP ==
  h_sub : Inport
  vel : Inport  Port=2
  lz : Inport  Port=3
  p : Inport  Port=4
  CD strut : Lookup_n-D  NumberOfTableDimensions=1  BreakpointsForDimension1=alpha0012  Table=cd0012  InternalRulePriority=Speed  RndMeth=Simplest
  Ddim : Product  Inputs=3
  Gain : Gain  Gain=0.5*rho*csF
  Gain1 : Gain  Gain=0.5
  Magnitude Squared : Math  Operator=magnitude^2
  Mpitch : Product
  Selector : Selector  InputPortWidth=3  IndexOptions=Index vector (dialog)  Indices=[1]  OutputSizes=1
  Selector1 : Selector  InputPortWidth=3  IndexOptions=Index vector (dialog)  Indices=[3]  OutputSizes=1
  Sum : Sum  Inputs=|-+
  a : Constant  Value=0
  a1 : Constant  Value=csF
  flip : Gain  Gain=-1
  lateralDamp : MATLAB Function  TreatAsAtomicUnit=on
  X : Outport
  K : Outport  Port=2
  M : Outport  Port=3
  wires:
  vel/1 -> Selector/1
  Selector/1 -> Magnitude Squared/1, lateralDamp/3(V)
  Magnitude Squared/1 -> Gain/1
  a/1 -> CD strut/1
  CD strut/1 -> Ddim/1
  Gain/1 -> Ddim/2
  h_sub/1 -> lateralDamp/1(h_sub), Ddim/3, Gain1/1
  Mpitch/1 -> M/1
  Gain1/1 -> Sum/1
  Sum/1 -> Mpitch/2
  Ddim/1 -> flip/1
  flip/1 -> Mpitch/1, X/1
  lz/1 -> Selector1/1
  Selector1/1 -> lateralDamp/2(zs), Sum/2
  a1/1 -> lateralDamp/5(cs)
  p/1 -> lateralDamp/4(p)
  lateralDamp/1(strutK) -> K/1

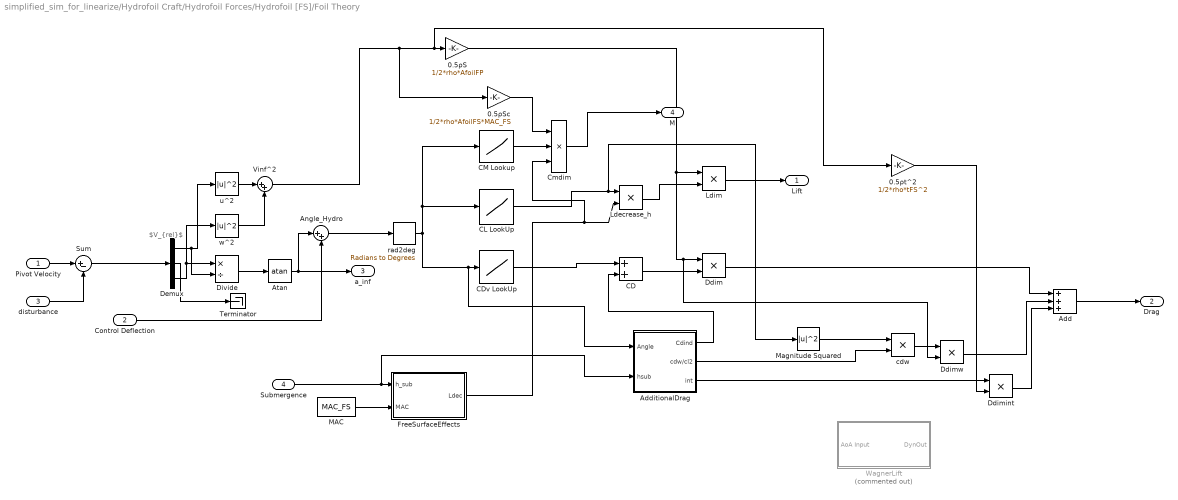
== system simplified_sim_for_linearize/Hydrofoil Craft/Hydrofoil Forces/Hydrofoil [FS]/Foil Theory ==
  note: $V_{rel}$
  Pivot Velocity : Inport
  Control Deflection : Inport  Port=2
  disturbance : Inport  Port=3
  Submergence : Inport  Port=4
  0.5ρS : Gain  Gain=1/2*rho*AfoilFP
  0.5ρSc : Gain  Gain=1/2*rho*AfoilFS*MAC_FS
  0.5ρt^2 : Gain  Gain=1/2*rho*tFS^2
  Add : Sum  Inputs=+++
  AdditionalDrag : Subsystem
  Angle_Hydro : Sum  Inputs=|++
  Atan : Trigonometry  Operator=atan
  CD : Sum
  CDv LookUp : Lookup_n-D  NumberOfTableDimensions=1  BreakpointsForDimension1=alpha63412wing  Table=cdv63412wing  InternalRulePriority=Speed  RndMeth=Simplest
  CL LookUp : Lookup_n-D  NumberOfTableDimensions=1  BreakpointsForDimension1=alpha63412wing  Table=cl63412wing  InternalRulePriority=Speed  RndMeth=Simplest
  CM Lookup : Lookup_n-D  NumberOfTableDimensions=1  BreakpointsForDimension1=alpha63412wing  Table=cm63412wing  InternalRulePriority=Speed  RndMeth=Simplest
  Cmdim : Product  Inputs=3
  Ddim : Product
  Ddimint : Product
  Ddimw : Product
  Demux : Demux  Outputs=3
  Divide : Product  Inputs=*/
  FreeSurfaceEffects : MATLAB Function  TreatAsAtomicUnit=on
  Ldecrease_h : Product
  Ldim : Product
  MAC : Constant  Value=MAC_FS
  Magnitude Squared : Math  Operator=magnitude^2
  Sum : Sum  Inputs=|+-
  Terminator : Terminator
  Vinf^2 : Sum  Inputs=|++
  WagnerLift : Subsystem  Commented=on
  cdw : Product
  rad2deg : simulink_extras/Transformations/Radians to Degrees
  u^2 : Math  Operator=magnitude^2
  w^2 : Math  Operator=magnitude^2
  Lift : Outport
  Drag : Outport  Port=2
  a_inf : Outport  Port=3
  M : Outport  Port=4
  wires:
  rad2deg/1 -> AdditionalDrag/1(Angle), CDv LookUp/1, CL LookUp/1, CM Lookup/1
  Demux/3 -> w^2/1, Divide/1
  Vinf^2/1 -> 0.5ρSc/1, 0.5ρt^2/1, 0.5ρS/1
  w^2/1 -> Vinf^2/2
  Demux/1 -> u^2/1, Divide/2
  Atan/1 -> a_inf/1, Angle_Hydro/1
  0.5ρS/1 -> Ddimw/2, Ddim/1, Ldim/1
  u^2/1 -> Vinf^2/1
  Divide/1 -> Atan/1
  Control Deflection/1 -> Angle_Hydro/2
  Demux/2 -> Terminator/1
  Ldim/1 -> Lift/1
  Sum/1 -> Demux/1
  disturbance/1 -> Sum/2
  Pivot Velocity/1 -> Sum/1
  Submergence/1 -> AdditionalDrag/2(hsub), FreeSurfaceEffects/1(h_sub)
  MAC/1 -> FreeSurfaceEffects/2(MAC)
  FreeSurfaceEffects/1(Ldec) -> Cmdim/3, Ldecrease_h/2
  CL LookUp/1 -> Magnitude Squared/1, Ldecrease_h/1
  Ldecrease_h/1 -> Ldim/2
  CDv LookUp/1 -> CD/1
  CD/1 -> Ddim/2
  AdditionalDrag/1(Cdind) -> CD/2
  Ddim/1 -> Add/1
  Magnitude Squared/1 -> cdw/1
  AdditionalDrag/2(cdw/cl2) -> cdw/2
  cdw/1 -> Ddimw/1
  Ddimw/1 -> Add/2
  AdditionalDrag/3(int) -> Ddimint/1
  Add/1 -> Drag/1
  0.5ρt^2/1 -> Ddimint/2
  Ddimint/1 -> Add/3
  Angle_Hydro/1 -> rad2deg/1
  CM Lookup/1 -> Cmdim/2
  0.5ρSc/1 -> Cmdim/1
  Cmdim/1 -> M/1

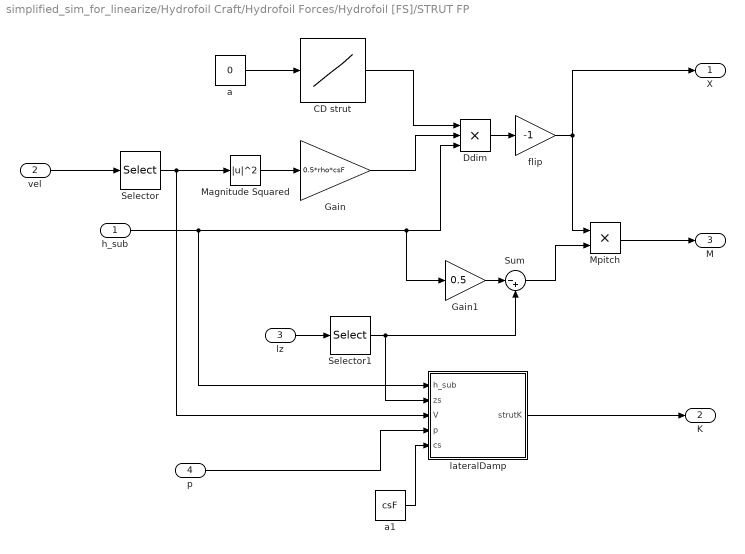
== system simplified_sim_for_linearize/Hydrofoil Craft/Hydrofoil Forces/Hydrofoil [FS]/STRUT FP ==
  h_sub : Inport
  vel : Inport  Port=2
  lz : Inport  Port=3
  p : Inport  Port=4
  CD strut : Lookup_n-D  NumberOfTableDimensions=1  BreakpointsForDimension1=alpha0012  Table=cd0012  InternalRulePriority=Speed  RndMeth=Simplest
  Ddim : Product  Inputs=3
  Gain : Gain  Gain=0.5*rho*csF
  Gain1 : Gain  Gain=0.5
  Magnitude Squared : Math  Operator=magnitude^2
  Mpitch : Product
  Selector : Selector  InputPortWidth=3  IndexOptions=Index vector (dialog)  Indices=[1]  OutputSizes=1
  Selector1 : Selector  InputPortWidth=3  IndexOptions=Index vector (dialog)  Indices=[3]  OutputSizes=1
  Sum : Sum  Inputs=|-+
  a : Constant  Value=0
  a1 : Constant  Value=csF
  flip : Gain  Gain=-1
  lateralDamp : MATLAB Function  TreatAsAtomicUnit=on
  X : Outport
  K : Outport  Port=2
  M : Outport  Port=3
  wires:
  vel/1 -> Selector/1
  Selector/1 -> Magnitude Squared/1, lateralDamp/3(V)
  Magnitude Squared/1 -> Gain/1
  a/1 -> CD strut/1
  CD strut/1 -> Ddim/1
  Gain/1 -> Ddim/2
  h_sub/1 -> lateralDamp/1(h_sub), Ddim/3, Gain1/1
  Mpitch/1 -> M/1
  Gain1/1 -> Sum/1
  Sum/1 -> Mpitch/2
  Ddim/1 -> flip/1
  flip/1 -> Mpitch/1, X/1
  lz/1 -> Selector1/1
  Selector1/1 -> lateralDamp/2(zs), Sum/2
  a1/1 -> lateralDamp/5(cs)
  p/1 -> lateralDamp/4(p)
  lateralDamp/1(strutK) -> K/1

== system simplified_sim_for_linearize/Hydrofoil Craft/Hydrofoil Forces/Hydrofoil [A]/Foil Theory/AdditionalDrag ==
  Angle : Inport
  hsub : Inport  Port=2
  Additional Drag : MATLAB Function  TreatAsAtomicUnit=on
  CD induced : Lookup_n-D  NumberOfTableDimensions=1  BreakpointsForDimension1=alpha63412wing  Table=cdi63412wing  InternalRulePriority=Speed  RndMeth=Simplest
  c : Constant  Value=MAC_A
  span : Constant  Value=spanA
  t : Constant  Value=tA
  Cdind : Outport
  cdw/cl2 : Outport  Port=2
  int : Outport  Port=3
  wires:
  Angle/1 -> CD induced/1
  CD induced/1 -> Additional Drag/1(cdind)
  Additional Drag/1(dinc) -> Cdind/1
  span/1 -> Additional Drag/2(span)
  hsub/1 -> Additional Drag/3(hsub)
  t/1 -> Additional Drag/4(t)
  c/1 -> Additional Drag/5(c)
  Additional Drag/2(cdw) -> cdw/cl2/1
  Additional Drag/3(cdint) -> int/1

== system simplified_sim_for_linearize/Hydrofoil Craft/Hydrofoil Forces/Hydrofoil [FP]/Foil Theory/AdditionalDrag ==
  Angle : Inport
  hsub : Inport  Port=2
  Additional Drag : MATLAB Function  TreatAsAtomicUnit=on
  CD induced : Lookup_n-D  NumberOfTableDimensions=1  BreakpointsForDimension1=alpha63412wing  Table=cdi63412wing  InternalRulePriority=Speed  RndMeth=Simplest
  c : Constant  Value=MAC_FP
  span : Constant  Value=spanFP
  t : Constant  Value=tFP
  Cdind : Outport
  cdw/cl2 : Outport  Port=2
  int : Outport  Port=3
  wires:
  Angle/1 -> CD induced/1
  CD induced/1 -> Additional Drag/1(cdind)
  Additional Drag/1(dinc) -> Cdind/1
  span/1 -> Additional Drag/2(span)
  hsub/1 -> Additional Drag/3(hsub)
  t/1 -> Additional Drag/4(t)
  c/1 -> Additional Drag/5(c)
  Additional Drag/2(cdw) -> cdw/cl2/1
  Additional Drag/3(cdint) -> int/1

== system simplified_sim_for_linearize/Hydrofoil Craft/Hydrofoil Forces/Hydrofoil [FS]/Foil Theory/AdditionalDrag ==
  Angle : Inport
  hsub : Inport  Port=2
  Additional Drag : MATLAB Function  TreatAsAtomicUnit=on
  CD induced : Lookup_n-D  NumberOfTableDimensions=1  BreakpointsForDimension1=alpha63412wing  Table=cdi63412wing  InternalRulePriority=Speed  RndMeth=Simplest
  c : Constant  Value=MAC_FS
  span : Constant  Value=spanFS
  t : Constant  Value=tFS
  Cdind : Outport
  cdw/cl2 : Outport  Port=2
  int : Outport  Port=3
  wires:
  Angle/1 -> CD induced/1
  CD induced/1 -> Additional Drag/1(cdind)
  Additional Drag/1(dinc) -> Cdind/1
  span/1 -> Additional Drag/2(span)
  hsub/1 -> Additional Drag/3(hsub)
  t/1 -> Additional Drag/4(t)
  c/1 -> Additional Drag/5(c)
  Additional Drag/2(cdw) -> cdw/cl2/1
  Additional Drag/3(cdint) -> int/1

== system simplified_sim_for_linearize/Hydrofoil Craft/Hydrofoil Forces/Hydrofoil [FS]/Foil Theory/WagnerLift ==
  AoA Input : Inport
  Add : Sum  Inputs=+++
  Gain : Gain  Gain=0.5
  wagn1 : TransferFcn  Numerator=[wagC1*wage1]  Denominator=[1 wage1]
  wagn2 : TransferFcn  Numerator=[wagC2*wage2]  Denominator=[1 wage2]
  DynOut : Outport
  wires:
  wagn1/1 -> Add/1
  AoA Input/1 -> wagn2/1, Gain/1, wagn1/1
  wagn2/1 -> Add/2
  Gain/1 -> Add/3
  Add/1 -> DynOut/1

== matlab function simplified_sim_for_linearize/Hydrofoil Craft/Hydrofoil Forces/Hydrofoil [A]/Foil Theory/FreeSurfaceEffects ==
  data: Ldec output; h_sub input; MAC input
function Ldec  = fcn(h_sub, MAC)

Ldec = 1 - 0.422*exp(-1.454*(h_sub/MAC));

== matlab function simplified_sim_for_linearize/Hydrofoil Craft/Hydrofoil Forces/Hydrofoil [FS]/CP ==
  data: lx output; ly output; ac input; lz output; foil_arm input
function [lx,ly,lz] = CP_HSF(ac, foil_arm)
% This function will calculate the moment arm for the center of 
% pressure of a hydrofoil based on control deflection. 
% Used when the pivot point is different from the center of pressure, and
% set to the original foil CP defined in the params otherwise.



lx = foil_arm(1);
ly = foil_arm(2);
lz = foil_arm(3);

== matlab function simplified_sim_for_linearize/Hydrofoil Craft/EOM/CRB MATRIX ==
  data: C output; nu input; M_RB parameter
% function CRB = CRBmatrix(uvw, pqr, mass, InertiaTensor, CG)
% 
% SMAT = @(x) [0 -x(3) x(2);
%             x(3) 0 -x(1);
%             -x(2) x(1) 0];
% CRB = [zeros(3,3), -mass*SMAT(uvw)-mass*SMAT(pqr)*SMAT(CG);
%         -mass*SMAT(uvw)+mass*SMAT(CG)*SMAT(pqr), -SMAT(InertiaTensor*pqr)];


function C = m2c(nu, M_RB)
M = M_RB;
% C = m2c(M,nu) computes the Coriolis-centripetal matrix C(nu) from the
% the system inertia matrix M > 0 for varying velocity nu. 
% If M is a 6x6 matrix and nu = [u, v, w, p, q, r]', the output is a 6x6 C matrix
% If M is a 3x3 matrix and nu = [u, v, r]', the output is a 3x3 C matrix.
%
% Examples: CRB = m2c(MRB,nu)     
%           CA  = m2c(MA, nu)
% Output:
%  C:  Coriolis-centripetal matrix C = C(nu) 
%
% Inputs:
%  M:  6x6 or 3x3 rigid-body MRB or added mass MA system marix 
%  nu: nu = [u, v, w, p, q, r]' or nu = [u, v, r]'
%
% The Coriolis and centripetal matrix depends on nu1 = [u,v,w]' and nu2 =
% [p,q,r]' as shown in Fossen (2021, Theorem 3.2). Alternatively, the matrix 
% CRB = CRB(nu2) can be computed using 
% 
% [MRB,CRB] = rbody(m,R44,R55,R66,nu2,r_bp) 
%
% which only requires the angular velocity vector nu2 = [p,q,r]'. This is 
% known as the linear velocity-independent representation.
%
% Author:    Thor I. Fossen
% Date:      14 Jun 2001
% Revisions: 26 Jun 2002, M21 = M12 is corrected to M12'
%            10 Jan 2004, the computation of C(nu) is generalized to a 
%                         nonsymmetric M > 0 (experimental data)
%            22 Oct 2020, generalized to accept 3-DOF horizontal-plane models
%            24 Apr 2021, updated the documentation

Smtrx = @(x) [0 -x(3) x(2);
             x(3) 0 -x(1);
            -x(2) x(1) 0];

M = 0.5 * (M + M');      % symmetrization of the inertia matrix

if (length(nu) == 6)     % 6-DOF model
     
    M11 = M(1:3,1:3);
    M12 = M(1:3,4:6);
    M21 = M12';
    M22 = M(4:6,4:6);

    nu1 = nu(1:3);
    nu2 = nu(4:6);
    nu1_dot = M11 * nu1 + M12 * nu2;
    nu2_dot = M21 * nu1 + M22 * nu2;

    C = [  zeros(3,3)      -Smtrx(nu1_dot)
          -Smtrx(nu1_dot)  -Smtrx(nu2_dot) ];
    
else   % 3-DOF model (surge, sway and yaw)
    
    C = [ 0                          0            -M(2,2)*nu(2)-M(2,3)*nu(3)
          0                          0             M(1,1)*nu(1)
          M(2,2)*nu(2)+M(2,3)*nu(3) -M(1,1)*nu(1)  0                      ];
    
end

== matlab function simplified_sim_for_linearize/Hydrofoil Craft/Hydrofoil Forces/Hydrofoil [FP]/Foil Theory/FreeSurfaceEffects ==
  data: Ldec output; h_sub input; MAC input
function Ldec  = fcn(h_sub, MAC)

Ldec = 1 - 0.422*exp(-1.454*(h_sub/MAC));

== matlab function simplified_sim_for_linearize/Hydrofoil Craft/Kinematics Equations ==
  data: euler_angles input size=3; uvw input size=3; pos_rates output size=3; pqr input size=3; euler_ang_rates output size=3
function [pos_rates, euler_ang_rates]= Kinematics(euler_angles, uvw, pqr)
    
phi = euler_angles(1);
theta = euler_angles(2);
psy = euler_angles(3);

DCM = [cos(psy)*cos(theta), -sin(psy)*cos(phi)+cos(psy)*sin(theta)*sin(phi), sin(psy)*sin(phi)+cos(psy)*cos(phi)*sin(theta);
    sin(psy)*cos(theta), cos(psy)*cos(phi)+sin(phi)*sin(theta)*sin(psy), -cos(psy)*sin(phi)+sin(theta)*sin(psy)*cos(phi);
    -sin(theta), sin(phi)*cos(theta), cos(theta)*cos(phi)];


attitudeMatrix = [1 sin(phi)*tan(theta) cos(phi)*tan(theta);
                  0 cos(phi) -sin(phi);
                  0 sin(phi)/cos(theta) cos(phi)/cos(theta)];

euler_ang_rates = attitudeMatrix*pqr;

pos_rates = DCM*uvw;

== matlab function simplified_sim_for_linearize/Hydrofoil Craft/Hydrofoil Forces/Hydrofoil [FS]/Foil Theory/AdditionalDrag/Additional Drag ==
  data: cdind input; dinc output; span input; hsub input; t input; c input; cdw output; cdint output; usted parameter
function [dinc, cdw, cdint]   = addedDrag(cdind, span, hsub, t, c, usted)

%V = 7m/s not very correct in general 
hsub = abs(hsub);
dinc = (2-(33*(hsub/span)^(3/2))/(33*(hsub/span)^(3/2)+1))*cdind;
frh = usted/sqrt(9.81*hsub);
cdw = 1/(2*frh^2)*(c/hsub)*exp(-2/frh^2);
cdint = 0.75*(t/c)-0.0003*(t/c)^(-2);

== matlab function simplified_sim_for_linearize/Hydrofoil Craft/Hydrofoil Forces/Hydrofoil [FS]/Foil Theory/FreeSurfaceEffects ==
  data: Ldec output; h_sub input; MAC input
function Ldec  = fcn(h_sub, MAC)

Ldec = 1 - 0.422*exp(-1.454*(h_sub/MAC));

== matlab function simplified_sim_for_linearize/Hydrofoil Craft/Hydrofoil Forces/Hydrofoil [A]/Force and Moment Calculation ==
  data: L input; D input; FX output; ainf input; FY output; FZ output; Marm input; MX output; MY output; MZ output
function [FX, FY, FZ, MX, MY, MZ] = HydrodynamicForces(L, D, ainf, Marm)


%%%%%%%%% ----------------- %%%%%%%%

% Vrel is :
% u+qz-ry  
% v+rx-pz
% w+py-qx

%Inflow velocity is this vector's magnitude, however, in 2D analysis,
%considering the y direction velocity will lead to issues. Change this if
%needed for lateral dynamics!

%Vinf_s is squared already
Rbh = [cos(ainf) 0 -sin(ainf);0 1 0;sin(ainf) 0 cos(ainf)];

forces = Rbh*[-D; 0; -L]; %Only Longitudinal Dynamics
[FX, FY, FZ] = deal(forces(1), forces(2), forces(3));
moments = cross(Marm,[FX, FY, FZ]);
[MX, MY, MZ] = deal(moments(1), moments(2), moments(3));

== matlab function simplified_sim_for_linearize/Hydrofoil Craft/Hydrofoil Forces/Hydrofoil [A]/STRUT FP/lateralDamp ==
  data: h_sub input; strutK output; zs input; V input; p input; cs input; rho parameter
function strutK = strutrolldamp(h_sub, zs, V, p, cs, rho)

strutK = -0.5*rho*V*2*pi*p*cs*(zs.^3-(zs+0.1-h_sub).^3)*(1/3);

== matlab function simplified_sim_for_linearize/Hydrofoil Craft/Hydrofoil Forces/Hydrofoil [FS]/Force and Moment Calculation ==
  data: L input; D input; FX output; ainf input; FY output; FZ output; Marm input; MX output; MY output; MZ output
function [FX, FY, FZ, MX, MY, MZ] = HydrodynamicForces(L, D, ainf, Marm)


%%%%%%%%% ----------------- %%%%%%%%

% Vrel is :
% u+qz-ry  
% v+rx-pz
% w+py-qx

%Inflow velocity is this vector's magnitude, however, in 2D analysis,
%considering the y direction velocity will lead to issues. Change this if
%needed for lateral dynamics!

%Vinf_s is squared already
Rbh = [cos(ainf) 0 -sin(ainf);0 1 0;sin(ainf) 0 cos(ainf)];

forces = Rbh*[-D; 0; -L]; %Only Longitudinal Dynamics
[FX, FY, FZ] = deal(forces(1), forces(2), forces(3));
moments = cross(Marm,[FX, FY, FZ]);
[MX, MY, MZ] = deal(moments(1), moments(2), moments(3));
